simulink subsystem "MM5"  (R2022b)
settings: Solver=VariableStepAuto  StartTime=0.0  StopTime=10.0  RelTol=1e-3
libraries: Raptor_lib x3
settings Model: Creator=serga  LastModifiedBy=serga

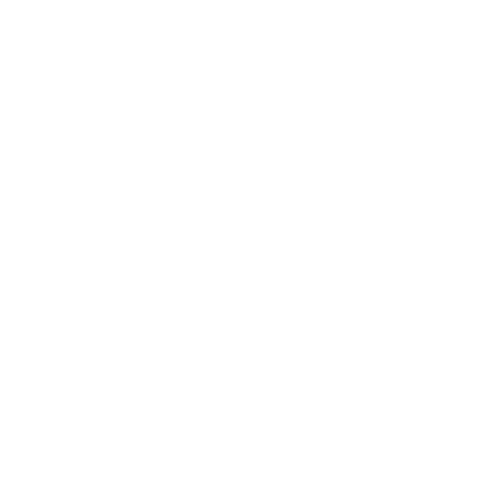
[thumbnail: Simulink's stored preview of the top-level diagram]
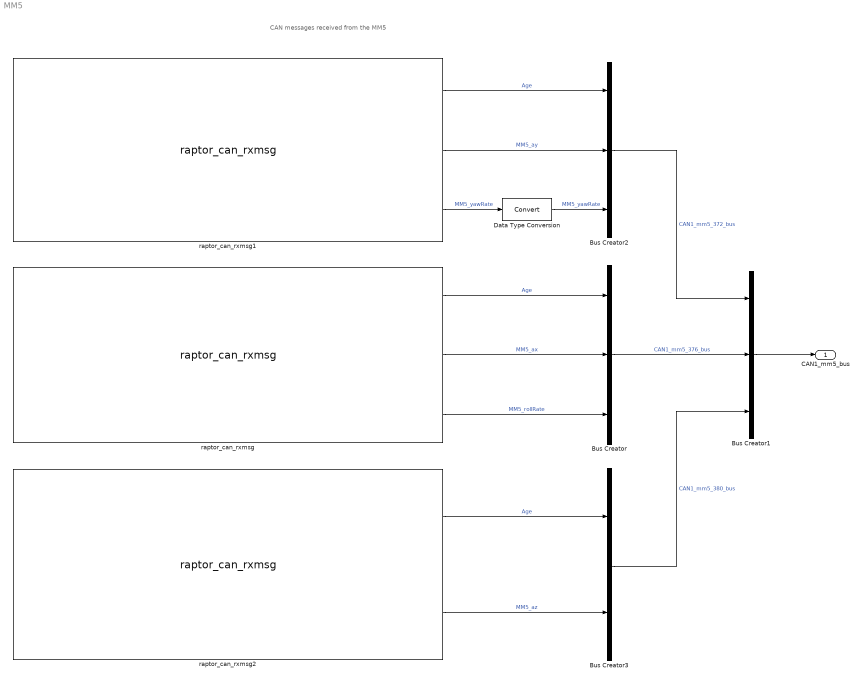
== system MM5 ==
  note: CAN messages received from the MM5
  Bus Creator : BusCreator  Inputs=3
  Bus Creator1 : BusCreator  Inputs=3
  Bus Creator2 : BusCreator  Inputs=3
  Bus Creator3 : BusCreator  Inputs=2
  Data Type Conversion : DataTypeConversion  SaturateOnIntegerOverflow=off  RndMeth=Floor
  raptor_can_rxmsg : Raptor_lib/CAN/raptor_can_rxmsg  canDefinition=struct('dbcFile', 'raptor_CAN1.dbc','message', 'MM5_376','comment', '','signals', {{'MM5_ax','MM5_rollRate'}},'enabled', [ 1 1;],'scaled', [ 1 1;],'canBus', '''CAN1''','messageID', [ 376;],'idMask', [ 536870911;],'payloadMask', [],'payloadValue', [],'period', [ 0;],'mailbox', '''''','queueSize', [ 1;],'label', [ 1;],'ver', [ 2;],'showID', [ 0;],'showRaw', [ 0;],'showRawMsg', [ 0;],'useStartVals', [ 0;],'extendedId', [ 0;],'showAge', [ 1;],'useSimFunc', [ 0;],'sim_func_name', '''''','fill', [ 0;],'editID', [ 0;],'signalOrder', [ 1;],'signalAscDes', [ 1;],'msgLength', [ 8;])  canBus='CAN1'  mailbox=''  payloadMask=[]  payloadValue=[]  idMask=hex2dec('1FFFFFFF')  queueSize=1  showID=0  label=1  fill=0  id=376  showRaw=0  showAge=1  signalOrder=1  signalInfo={{struct('Name', 'MM5_rollRate','StartBit', [ 0;],'SignalSize', [ 16;],'ByteOrder', 'LittleEndian','ValueType', 'UNSIGNED','Class', 'uint16','Signed', [ 0;],'Factor', [ -0.005;],'Offset', [ 163.9;],'Min', [ -100;],'Max', [ 100;],'Units', '','StartVal', [ 0;],'Comment', 'Roll Rate','Multiplexed', [ 0;],'Multiplexor', [ 0;],'MultiplexMode_Min', [ 0;],'MultiplexMode_Max', [ 0;]),struct('Name', 'MM5_ax','StartBit', [ 32;],'SignalSize', [ 16;],'ByteOrder', 'LittleEndian','ValueType', 'UNSIGNED','Class', 'uint16','Signed', [ 0;],'Factor', [ -0.0001274;],'Offset', [ 4.1746;],'Min', [ -100;],'Max', [ 100;],'Units', '','StartVal', [ 0;],'Comment', 'Acceleration X Axis','Multiplexed', [ 0;],'Multiplexor', [ 0;],'MultiplexMode_Min', [ 0;],'MultiplexMode_Max', [ 0;])}}  showRawMsg=0  useSimFunc=0  sim_func_name=''  useStartVals=0  extendedId=0
      settings: SourceProductName=Raptor
  raptor_can_rxmsg1 : Raptor_lib/CAN/raptor_can_rxmsg  canDefinition=struct('dbcFile', 'raptor_CAN1.dbc','message', 'MM5_372','comment', '','signals', {{'MM5_ay','MM5_yawRate'}},'enabled', [ 1 1;],'scaled', [ 1 1;],'canBus', '''CAN1''','messageID', [ 372;],'idMask', [ 536870911;],'payloadMask', [],'payloadValue', [],'period', [ 0;],'mailbox', '''''','queueSize', [ 1;],'label', [ 1;],'ver', [ 2;],'showID', [ 0;],'showRaw', [ 0;],'showRawMsg', [ 0;],'useStartVals', [ 0;],'extendedId', [ 0;],'showAge', [ 1;],'useSimFunc', [ 0;],'sim_func_name', '''''','fill', [ 0;],'editID', [ 0;],'signalOrder', [ 1;],'signalAscDes', [ 1;],'msgLength', [ 8;])  canBus='CAN1'  mailbox=''  payloadMask=[]  payloadValue=[]  idMask=hex2dec('1FFFFFFF')  queueSize=1  showID=0  label=1  fill=0  id=372  showRaw=0  showAge=1  signalOrder=1  signalInfo={{struct('Name', 'MM5_yawRate','StartBit', [ 0;],'SignalSize', [ 16;],'ByteOrder', 'LittleEndian','ValueType', 'UNSIGNED','Class', 'uint16','Signed', [ 0;],'Factor', [ 0.005;],'Offset', [ -163.9;],'Min', [ -100;],'Max', [ 100;],'Units', '','StartVal', [ 0;],'Comment', 'Yaw Rate','Multiplexed', [ 0;],'Multiplexor', [ 0;],'MultiplexMode_Min', [ 0;],'MultiplexMode_Max', [ 0;]),struct('Name', 'MM5_ay','StartBit', [ 32;],'SignalSize', [ 16;],'ByteOrder', 'LittleEndian','ValueType', 'UNSIGNED','Class', 'uint16','Signed', [ 0;],'Factor', [ -0.0001274;],'Offset', [ 4.1746;],'Min', [ -100;],'Max', [ 100;],'Units', '','StartVal', [ 0;],'Comment', 'Acceleration Y Axis','Multiplexed', [ 0;],'Multiplexor', [ 0;],'MultiplexMode_Min', [ 0;],'MultiplexMode_Max', [ 0;])}}  showRawMsg=0  useSimFunc=0  sim_func_name=''  useStartVals=0  extendedId=0
      settings: SourceProductName=Raptor
  raptor_can_rxmsg2 : Raptor_lib/CAN/raptor_can_rxmsg  canDefinition=struct('dbcFile', 'raptor_CAN1.dbc','message', 'MM5_380','comment', '','signals', {{'MM5_az'}},'enabled', [ 1;],'scaled', [ 1;],'canBus', '''CAN1''','messageID', [ 380;],'idMask', [ 536870911;],'payloadMask', [],'payloadValue', [],'period', [ 0;],'mailbox', '''''','queueSize', [ 1;],'label', [ 1;],'ver', [ 2;],'showID', [ 0;],'showRaw', [ 0;],'showRawMsg', [ 0;],'useStartVals', [ 0;],'extendedId', [ 0;],'showAge', [ 1;],'useSimFunc', [ 0;],'sim_func_name', '''''','fill', [ 0;],'editID', [ 0;],'signalOrder', [ 1;],'signalAscDes', [ 1;],'msgLength', [ 8;])  canBus='CAN1'  mailbox=''  payloadMask=[]  payloadValue=[]  idMask=hex2dec('1FFFFFFF')  queueSize=1  showID=0  label=1  fill=0  id=380  showRaw=0  showAge=1  signalOrder=1  signalInfo={{struct('Name', 'MM5_az','StartBit', [ 32;],'SignalSize', [ 16;],'ByteOrder', 'LittleEndian','ValueType', 'UNSIGNED','Class', 'uint16','Signed', [ 0;],'Factor', [ -0.0001274;],'Offset', [ 4.1746;],'Min', [ -100;],'Max', [ 100;],'Units', '','StartVal', [ 0;],'Comment', 'Acceleration Z Axis','Multiplexed', [ 0;],'Multiplexor', [ 0;],'MultiplexMode_Min', [ 0;],'MultiplexMode_Max', [ 0;])}}  showRawMsg=0  useSimFunc=0  sim_func_name=''  useStartVals=0  extendedId=0
      settings: SourceProductName=Raptor
  CAN1_mm5_bus : Outport
  wires:
  Data Type Conversion/1 -> Bus Creator2/3  "MM5_yawRate"
  Bus Creator1/1 -> CAN1_mm5_bus/1
  raptor_can_rxmsg1/3 -> Data Type Conversion/1  "MM5_yawRate"
  raptor_can_rxmsg1/2 -> Bus Creator2/2  "MM5_ay"
  raptor_can_rxmsg1/1 -> Bus Creator2/1  "Age"
  raptor_can_rxmsg/1 -> Bus Creator/1  "Age"
  raptor_can_rxmsg/2 -> Bus Creator/2  "MM5_ax"
  raptor_can_rxmsg/3 -> Bus Creator/3  "MM5_rollRate"
  raptor_can_rxmsg2/2 -> Bus Creator3/2  "MM5_az"
  raptor_can_rxmsg2/1 -> Bus Creator3/1  "Age"
  Bus Creator2/1 -> Bus Creator1/1  "CAN1_mm5_372_bus"
  Bus Creator/1 -> Bus Creator1/2  "CAN1_mm5_376_bus"
  Bus Creator3/1 -> Bus Creator1/3  "CAN1_mm5_380_bus"
